simulink model "mujoco_withController"  (R2023b)
settings: Solver=VariableStepAuto  StartTime=0.0  StopTime=150  RelTol=1e-3
libraries: robotcorelib x1, vrlib x1, mjLib x1
settings Model: Creator=omer  LastModifiedBy=omer
settings OptimizationCC: ReuseModelBlockBuffer=off

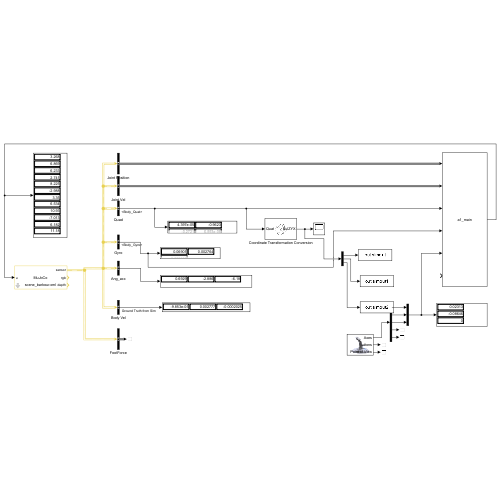
[thumbnail: Simulink's stored preview of the top-level diagram]
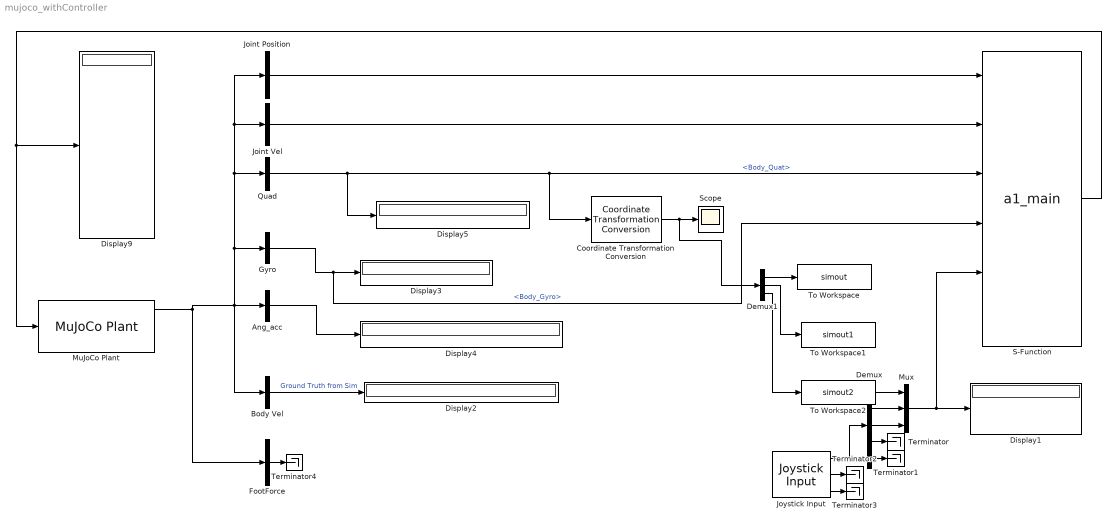
== system mujoco_withController ==
  Ang_acc : BusSelector  OutputSignals=Body_Acc  OutputAsBus=on
  Body Vel : BusSelector  OutputSignals=Body_Vel_velocimeter  OutputAsBus=on
  Coordinate Transformation Conversion : robotcorelib/Coordinate Transformation Conversion  InputRepresentation=Quaternion  InputEulerSequence=ZYX  ShowTrVecInputPort=on  OutputRepresentation=Euler Angles  OutputEulerSequence=ZYX  ShowTrVecOutputPort=on  SimulateUsing=Interpreted execution
  Demux : Demux  Outputs=5
  Demux1 : Demux  Outputs=3
  Display{1..5,9} (6 alike) : Display
  FootForce : BusSelector  OutputSignals=FR_footForce,FL_footForce,RR_footForce,RL_footForce  OutputAsBus=on
  Gyro : BusSelector  OutputSignals=Body_Gyro
  Joint Position : BusSelector  OutputSignals=FR_hip_pos,FR_thigh_pos,FR_calf_pos,FL_hip_pos,FL_thigh_pos,FL_calf_pos,RR_hip_pos,RR_thigh_pos,RR_calf_pos,RL_hip_pos,RL_thigh_pos,RL_calf_pos  OutputAsBus=on
  Joint Vel : BusSelector  OutputSignals=FR_hip_vel,FR_thigh_vel,FR_calf_vel,FL_hip_vel,FL_thigh_vel,FL_calf_vel,RR_hip_vel,RR_thigh_vel,RR_calf_vel,RL_hip_vel,RL_thigh_vel,RL_calf_vel  OutputAsBus=on
  Joystick Input : vrlib/Joystick Input  joyid=1  adjustports=on  forcefeed=off
  MuJoCo Plant : mjLib/MuJoCo Plant  controlBus=[]  sensorBus=mj_bus_sensor_7979902499018342666  controlLength=[]  sensorLength=[]  rgbLength=[]  depthLength=[]  sampleTime=0.001  xmlFileRel=C:\Users\omer\Desktop\MyQuadruped\model\barkour_a1_old\scene_barkour.xml  xmlFile=C:\Users\omer\Desktop\MyQuadruped\model\barkour_a1_old\scene_barkour.xml  renderingType=Global  vsync=off  visualFPS=60  zoomLevel=1  znear=0.22627  zfar=1131.371  cameraSampleTime=0.020  rgbOutOption=on  depthOutOption=on  controlInterfaceType=Vector
      settings: SourceProductName=MuJoCo Simulator
  Mux : Mux  Inputs=3
  Quad : BusSelector  OutputSignals=Body_Quat
  S-Function : S-Function  FunctionName=a1_main  SFunctionDeploymentMode=off  EnableBusSupport=off
  Scope : Scope
  Terminator{,1..4} (5 alike) : Terminator
  To Workspace : ToWorkspace  VariableName=simout  SaveFormat=Timeseries  SampleTime=-1
  To Workspace1 : ToWorkspace  VariableName=simout1  SaveFormat=Timeseries  SampleTime=-1
  To Workspace2 : ToWorkspace  VariableName=simout2  SaveFormat=Timeseries  SampleTime=-1
  wires:
  S-Function/1 -> Display9/1, MuJoCo Plant/1
  Quad/1 -> Display5/1, Coordinate Transformation Conversion/1, S-Function/3  "<Body_Quat>"
  Demux/1 -> Mux/1
  Demux/2 -> Mux/2
  Demux/3 -> Mux/3
  Demux/4 -> Terminator/1
  Demux/5 -> Terminator1/1
  Joystick Input/1 -> Demux/1
  Joystick Input/2 -> Terminator2/1
  Body Vel/1 -> Display2/1  "Ground Truth from Sim"
  Gyro/1 -> S-Function/4, Display3/1  "<Body_Gyro>"
  Ang_acc/1 -> Display4/1
  MuJoCo Plant/1 -> Body Vel/1, Ang_acc/1, Gyro/1, Joint Vel/1, Joint Position/1, Quad/1, FootForce/1
  Joint Position/1 -> S-Function/1
  Joint Vel/1 -> S-Function/2
  FootForce/1 -> Terminator4/1
  Joystick Input/3 -> Terminator3/1
  Mux/1 -> S-Function/5, Display1/1
  Demux1/1 -> To Workspace/1
  Coordinate Transformation Conversion/1 -> Demux1/1, Scope/1
  Demux1/2 -> To Workspace1/1
  Demux1/3 -> To Workspace2/1
